simulink library "Stimulation_Currents_lib"  (Simulink 6.2)
settings Model: LastModifiedBy=bsaunder  ExtModeAutoUpdateStatusClock=off

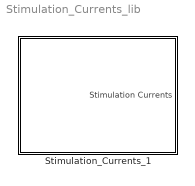
== system Stimulation_Currents_lib ==
  Stimulation_Currents_1 : Subsystem  mask(StimCurrentInput){Quad_R=110, Ham_R=80, Glut_R=80, Calf_R=0, ExactOpp=on, Quad_L=[110], Ham_L=[80], Glut_L=[80], Calf_L=[0]}
      mask prompts: Quad_R "Quad. Right"; Ham_R "Ham. Right"; Glut_R "Glut. Right"; Calf_R "Calf Right"; ExactOpp "Force left leg to use the same current as the right leg"; Quad_L "Quad. Left"; Ham_L "Ham. Left"; Glut_L "Glut. Left"; Calf_L "Calf Left"
      mask help: Use this block to input the stimulation currents. Currents should be in mA. Output is an 8 element bus vector.
      mask init:
      | if ExactOpp
      |   Quad_L = Quad_R;
      |   set_param(gcb, 'Quad_L', ['[',num2str(Quad_L),']']);
      | 
      |   Ham_L = Ham_R;
      |   set_param(gcb, 'Ham_L', ['[',num2str(Ham_L),']']);
      | 
      |   Glut_L = Glut_R;
      |   set_param(gcb, 'Glut_L', ['[',num2str(Glut_L),']']);
      | 
      |   Calf_L = Calf_R;
      |   set_param(gcb, 'Calf_L', ['[',num2str(Calf_L),']']);
      | end
      mask CallbackString:
      | ||||if strcmp(get_param(gcb,'ExactOpp'),'on')
      | set_param(gcb,'MaskVisibilities', {'on', 'on', 'on', 'on', 'on', 'off', 'off', 'off', 'off'});
      | else
      | set_param(gcb,'MaskVisibilities', {'on', 'on', 'on', 'on', 'on', 'on', 'on', 'on', 'on'});
      | end
      | ||||
      mask Display:
      | text(0.5, 0.9, 'Stimulation Current', 'HorizontalAlignment', 'center', 'VerticalAlignment', 'middle');
      | 
      | plot([0.05 0.95], [0.65 0.65]);
      | plot([0.35 0.35], [0.8 0.2]);
      | plot([0.65 0.65], [0.8 0.2]);
      | 
      | text(0.2, 0.7, 'Muscle', 'HorizontalAlignment', 'center', 'VerticalAlignment', 'middle');
      | text(0.5, 0.7, 'Right', 'HorizontalAlignment', 'center', 'VerticalAlignment', 'middle');
      | text(0.8, 0.7, 'Left', 'HorizontalAlignment', 'center', 'VerticalAlignment', 'middle');
      | 
      | text(0.2, 0.55, 'Q', 'HorizontalAlignment', 'center', 'VerticalAlignment', 'middle');
      | text(0.5, 0.55, num2str(Quad_R), 'HorizontalAlignment', 'center', 'VerticalAlignment', 'middle');
      | text(0.8, 0.55, num2str(Quad_L), 'HorizontalAlignment', 'center', 'VerticalAlignment', 'middle');
      | 
      | text(0.2, 0.45, 'H', 'HorizontalAlignment', 'center', 'VerticalAlignment', 'middle');
      | text(0.5, 0.45, num2str(Ham_R), 'HorizontalAlignment', 'center', 'VerticalAlignment', 'middle');
      | text(0.8, 0.45, num2str(Ham_L), 'HorizontalAlignment', 'center', 'VerticalAlignment', 'middle');
      | 
      | text(0.2, 0.35, 'G', 'HorizontalAlignment', 'center', 'VerticalAlignment', 'middle');
      | text(0.5, 0.35, num2str(Glut_R), 'HorizontalAlignment', 'center', 'VerticalAlignment', 'middle');
      | text(0.8, 0.35, num2str(Glut_L), 'HorizontalAlignment', 'center', 'VerticalAlignment', 'middle');
      | 
      | text(0.2, 0.25, 'C', 'HorizontalAlignment', 'center', 'VerticalAlignment', 'middle');
      | text(0.5, 0.25, num2str(Calf_R), 'HorizontalAlignment', 'center', 'VerticalAlignment', 'middle');
      | text(0.8, 0.25, num2str(Calf_L), 'HorizontalAlignment', 'center', 'VerticalAlignment', 'middle');

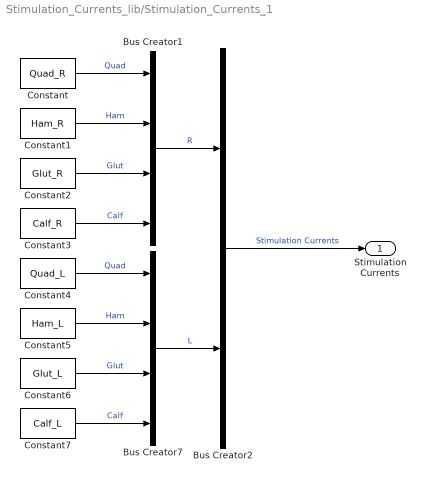
== system Stimulation_Currents_lib/Stimulation_Currents_1 ==
  Bus Creator1 : BusCreator
  Bus Creator2 : BusCreator  Inputs=2
  Bus Creator7 : BusCreator
  Constant : Constant  Value=Quad_R
  Constant1 : Constant  Value=Ham_R
  Constant2 : Constant  Value=Glut_R
  Constant3 : Constant  Value=Calf_R
  Constant4 : Constant  Value=Quad_L
  Constant5 : Constant  Value=Ham_L
  Constant6 : Constant  Value=Glut_L
  Constant7 : Constant  Value=Calf_L
  Stimulation Currents : Outport
  wires:
  Constant7/1 -> Bus Creator7/4  "Calf"
  Constant6/1 -> Bus Creator7/3  "Glut"
  Constant5/1 -> Bus Creator7/2  "Ham"
  Constant4/1 -> Bus Creator7/1  "Quad"
  Constant3/1 -> Bus Creator1/4  "Calf"
  Constant2/1 -> Bus Creator1/3  "Glut"
  Constant1/1 -> Bus Creator1/2  "Ham"
  Constant/1 -> Bus Creator1/1  "Quad"
  Bus Creator1/1 -> Bus Creator2/1  "R"
  Bus Creator7/1 -> Bus Creator2/2  "L"
  Bus Creator2/1 -> Stimulation Currents/1  "Stimulation Currents"
